simulink model "Template"  (Simulink 7.3)
settings: Solver=ode45  StartTime=0.0  StopTime=10.0  RelTol=1e-3
libraries: marine_gnc x4, dspmtrx3 x2, simulink x2, simulink_extras x1
settings Model: Creator=mcl  LastModifiedBy=mcl

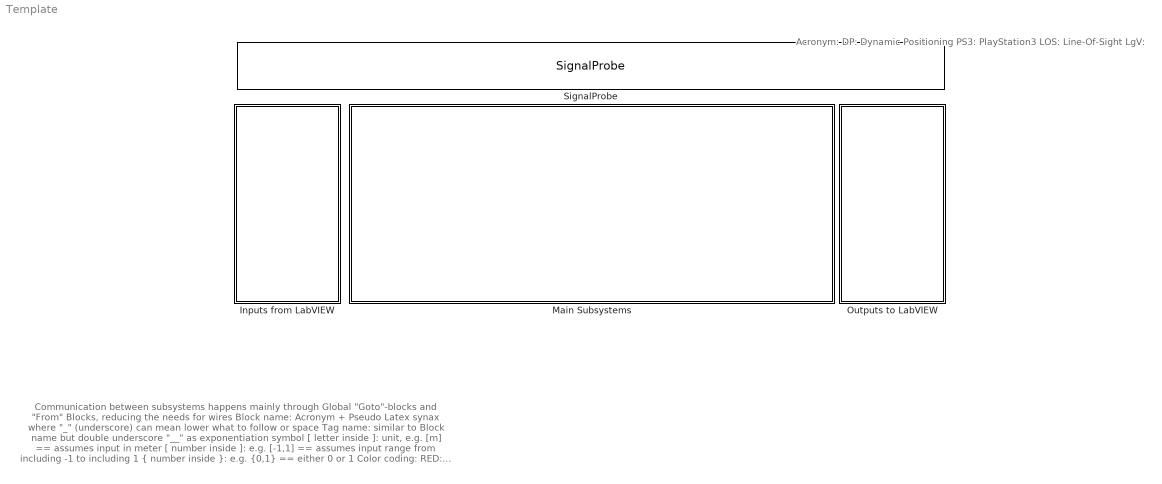
== system Template ==
  note: Communication between subsystems happens mainly through Global "Goto"-blocks and "From" Blocks,
      | reducing the needs for wires
      |
      | Block name: Acronym + Pseudo Latex synax where "_" (underscore) can mean lower what to follow or space
      | Tag name: similar to Block name but double underscore "__" as exponentiation symbol
      |
      | [ letter inside ]: unit, e.g. [m] == assumes input in meter
      | [ number inside ]: e.g. [-1,1] == assumes input range from including -1 to including 1
      | { number inside }:  e.g. {0,1} == either 0 or 1
      |
      | Color coding:
      | RED: Sinks (output ports, terminators, to workspace blocks, etc.)
      | GREEN Sources (inputs ports, constants, etc.)
      | CYAN: Memory blocks: Integrators, unit delays, memory, transfer functions, state space blocks, etc
      | GRAY: Logics blocks: Logic action ports, subsystem enable, etc.
      | ORANGE: GOTO blocks
      | MAGENTA: FROM blocks
      | YELLOW: All remaining blocks,
  note: Acronym:
      | DP: Dynamic Positioning
      | PS3: PlayStation3
      | LOS: Line-Of-Sight
      | LgV:
  Inputs from LabVIEW : Subsystem
  Main Subsystems : Subsystem
  Outputs to LabVIEW : Subsystem
  SignalProbe : S-Function  Description=Use this block with SIT.  FunctionName=SignalProbe  Parameters=1  EnableBusSupport=off
      settings: PreSaveFcn=NISIT_ModelVars;
      mask Description: The LabVIEW Simulation Interface Toolkit uses the SignalProbe block to probe the signals in the model. The SignalProbe block must be on the top level of the model hierarchy. You can have only one SignalProbe block per model file. Do not rename the SignalProbe block. Do not change the name of another model block to SignalProbe.

== system Template/Inputs from LabVIEW ==
  Control Input Selector : Constant  Value=0
  Control Mode Selector : Constant  Value=0
  DynamicPositioning : Subsystem
  Enable CSE1 : Constant  Value=0
  Initial eta : Subsystem
  Initial nu : Subsystem
  LOS LgV backstepping II : Subsystem
  Linear Simulator : Subsystem
  Path : Subsystem
  PlayStation3 : Subsystem
  tag scope: Control_Input_Selector=global, Control_Mode_Selector=global, Enable_CSE1=global
  wires:
  Control Mode Selector/1 -> [Control_Mode_Selector]
  Control Input Selector/1 -> [Control_Input_Selector]
  Enable CSE1/1 -> [Enable_CSE1]

== system Template/Main Subsystems ==
  DP control : Subsystem
  Guidance : Subsystem
  Input from SIT : Subsystem
  Subsystem : Subsystem

== system Template/Outputs to LabVIEW ==
  note: Gain blocks in this subsystem, functions as output ports for linking LabVIEW indicators through SIT Connection Manager
  Battery Voltage : Subsystem

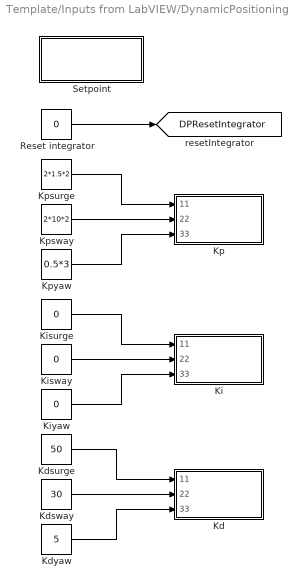
== system Template/Inputs from LabVIEW/DynamicPositioning ==
  Kd : Subsystem
  Kdsurge : Constant  Value=50
  Kdsway : Constant  Value=30
  Kdyaw : Constant  Value=5
  Ki : Subsystem
  Kisurge : Constant  Value=0
  Kisway : Constant  Value=0
  Kiyaw : Constant  Value=0
  Kp : Subsystem
  Kpsurge : Constant  Value=2*1.5*2
  Kpsway : Constant  Value=2*10*2
  Kpyaw : Constant  Value=0.5*3
  Reset integrator : Constant  Value=0
  Setpoint : Subsystem
  tag scope: DPResetIntegrator=global
  wires:
  Reset integrator/1 -> [DPResetIntegrator]
  Kpsurge/1 -> Kp/1(11)
  Kpsway/1 -> Kp/2(22)
  Kpyaw/1 -> Kp/3(33)
  Kdsurge/1 -> Kd/1(11)
  Kdsway/1 -> Kd/2(22)
  Kdyaw/1 -> Kd/3(33)
  Kisurge/1 -> Ki/1(11)
  Kisway/1 -> Ki/2(22)
  Kiyaw/1 -> Ki/3(33)

== system Template/Inputs from LabVIEW/Initial eta ==
  Mux : Mux  Inputs=3
  psi_0 : Constant  Value=0  OutDataType=fixdt(1, 16)  OutScaling=2^0
  x_0 : Constant  Value=0  OutDataType=fixdt(1, 16)  OutScaling=2^0
  y_0 : Constant  Value=0  OutDataType=fixdt(1, 16)  OutScaling=2^0
  eta_0 : Outport  OutDataType=fixdt(1, 16)  OutScaling=2^0
  wires:
  x_0/1 -> Mux/1
  y_0/1 -> Mux/2
  psi_0/1 -> Mux/3
  Mux/1 -> eta_0/1

== system Template/Inputs from LabVIEW/Initial nu ==
  Mux : Mux  Inputs=3
  r_0 : Constant  Value=0  OutDataType=fixdt(1, 16)  OutScaling=2^0
  u_0 : Constant  Value=0  OutDataType=fixdt(1, 16)  OutScaling=2^0
  v_0 : Constant  Value=0  OutDataType=fixdt(1, 16)  OutScaling=2^0
  nu_0 : Outport  OutDataType=fixdt(1, 16)  OutScaling=2^0
  wires:
  u_0/1 -> Mux/1
  v_0/1 -> Mux/2
  r_0/1 -> Mux/3
  Mux/1 -> nu_0/1

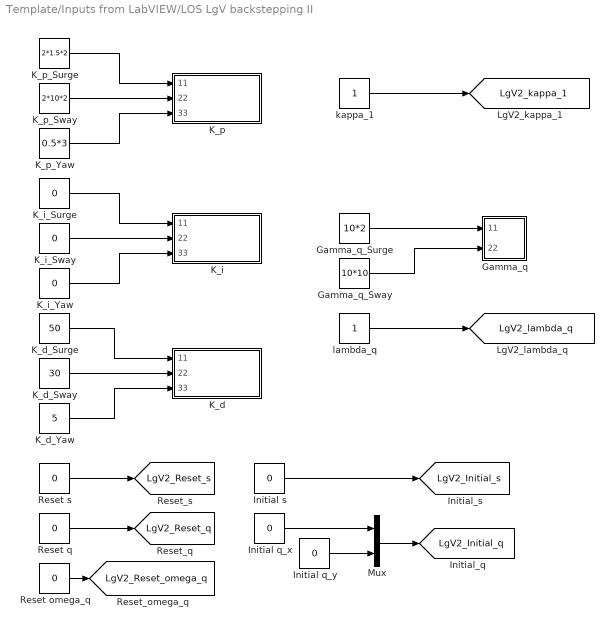
== system Template/Inputs from LabVIEW/LOS LgV backstepping II ==
  Gamma_q : Subsystem
  Gamma_q_Surge : Constant  Value=10*2
  Gamma_q_Sway : Constant  Value=10*10
  Initial q_x : Constant  Value=0  OutDataType=fixdt(1, 16)  OutScaling=2^0
  Initial q_y : Constant  Value=0  OutDataType=fixdt(1, 16)  OutScaling=2^0
  Initial s : Constant  Value=0  OutDataType=fixdt(1, 16)  OutScaling=2^0
  K_d : Subsystem
  K_d_Surge : Constant  Value=50
  K_d_Sway : Constant  Value=30
  K_d_Yaw : Constant  Value=5
  K_i : Subsystem
  K_i_Surge : Constant  Value=0
  K_i_Sway : Constant  Value=0
  K_i_Yaw : Constant  Value=0
  K_p : Subsystem
  K_p_Surge : Constant  Value=2*1.5*2
  K_p_Sway : Constant  Value=2*10*2
  K_p_Yaw : Constant  Value=0.5*3
  Mux : Mux  Inputs=2
  Reset omega_q : Constant  Value=0
  Reset q : Constant  Value=0
  Reset s : Constant  Value=0
  kappa_1 : Constant
  lambda_q : Constant
  tag scope: LgV2_Initial_q=global, LgV2_Initial_s=global, LgV2_Reset_omega_q=global, LgV2_Reset_q=global, LgV2_Reset_s=global, LgV2_kappa_1=global, LgV2_lambda_q=global
  wires:
  K_p_Surge/1 -> K_p/1(11)
  K_p_Sway/1 -> K_p/2(22)
  K_p_Yaw/1 -> K_p/3(33)
  K_d_Surge/1 -> K_d/1(11)
  K_d_Sway/1 -> K_d/2(22)
  K_d_Yaw/1 -> K_d/3(33)
  K_i_Surge/1 -> K_i/1(11)
  K_i_Sway/1 -> K_i/2(22)
  K_i_Yaw/1 -> K_i/3(33)
  Gamma_q_Surge/1 -> Gamma_q/1(11)
  Gamma_q_Sway/1 -> Gamma_q/2(22)
  kappa_1/1 -> [LgV2_kappa_1]
  lambda_q/1 -> [LgV2_lambda_q]
  Initial q_x/1 -> Mux/1
  Initial q_y/1 -> Mux/2
  Reset s/1 -> [LgV2_Reset_s]
  Reset q/1 -> [LgV2_Reset_q]
  Initial s/1 -> [LgV2_Initial_s]
  Mux/1 -> [LgV2_Initial_q]
  Reset omega_q/1 -> [LgV2_Reset_omega_q]

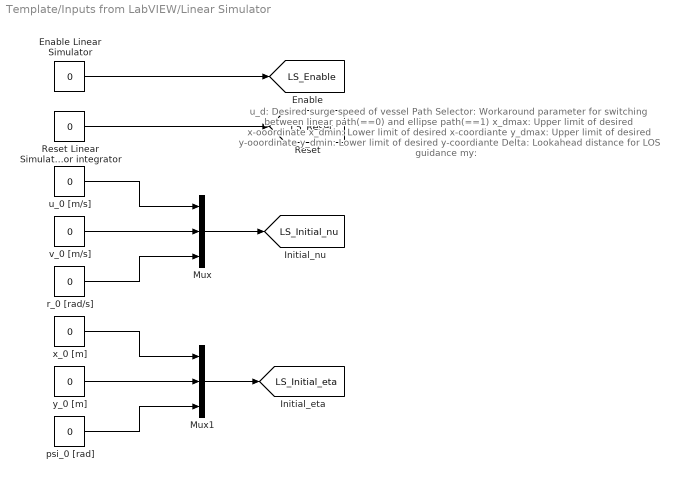
== system Template/Inputs from LabVIEW/Linear Simulator ==
  note: u_d: Desired surge speed of vessel
      | Path Selector: Workaround parameter for switching between linear path(==0) and ellipse path(==1)
      | x_dmax: Upper limit of desired x-ooordinate
      | x_dmin: Lower limit of desired x-coordiante
      | y_dmax: Upper limit of desired y-ooordinate
      | y_dmin: Lower limit of desired y-coordiante
      | Delta: Lookahead distance for LOS guidance
      | my:
  Enable Linear Simulator : Constant  Value=0
  Mux : Mux  Inputs=3
  Mux1 : Mux  Inputs=3
  Reset Linear Simulator integrator : Constant  Value=0
  psi_0 [rad] : Constant  Value=0  OutDataType=fixdt(1, 16)  OutScaling=2^0
  r_0 [rad/s] : Constant  Value=0  OutDataType=fixdt(1, 16)  OutScaling=2^0
  u_0 [m/s] : Constant  Value=0  OutDataType=fixdt(1, 16)  OutScaling=2^0
  v_0 [m/s] : Constant  Value=0  OutDataType=fixdt(1, 16)  OutScaling=2^0
  x_0 [m] : Constant  Value=0  OutDataType=fixdt(1, 16)  OutScaling=2^0
  y_0 [m] : Constant  Value=0  OutDataType=fixdt(1, 16)  OutScaling=2^0
  tag scope: LS_Enable=global, LS_Initial_eta=global, LS_Initial_nu=global, LS_Reset=global
  wires:
  Enable Linear Simulator/1 -> [LS_Enable]
  Reset Linear Simulator integrator/1 -> [LS_Reset]
  Mux/1 -> [LS_Initial_nu]
  r_0 [rad/s]/1 -> Mux/3
  v_0 [m/s]/1 -> Mux/2
  u_0 [m/s]/1 -> Mux/1
  Mux1/1 -> [LS_Initial_eta]
  psi_0 [rad]/1 -> Mux1/3
  y_0 [m]/1 -> Mux1/2
  x_0 [m]/1 -> Mux1/1

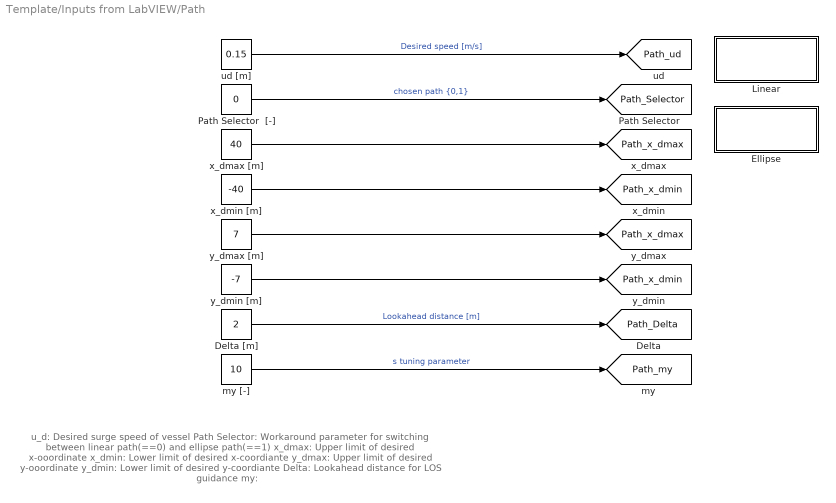
== system Template/Inputs from LabVIEW/Path ==
  note: u_d: Desired surge speed of vessel
      | Path Selector: Workaround parameter for switching between linear path(==0) and ellipse path(==1)
      | x_dmax: Upper limit of desired x-ooordinate
      | x_dmin: Lower limit of desired x-coordiante
      | y_dmax: Upper limit of desired y-ooordinate
      | y_dmin: Lower limit of desired y-coordiante
      | Delta: Lookahead distance for LOS guidance
      | my:
  Delta [m] : Constant  Value=2  OutDataType=fixdt(1, 16)  OutScaling=2^0
  Ellipse : Subsystem
  Linear : Subsystem
  Path Selector  [-] : Constant  Value=0
  my [-] : Constant  Value=10  OutDataType=fixdt(1, 16)  OutScaling=2^0
  ud [m] : Constant  Value=0.15  OutDataType=fixdt(1, 16)  OutScaling=2^0
  x_dmax [m] : Constant  Value=40
  x_dmin [m] : Constant  Value=-40
  y_dmax [m] : Constant  Value=7
  y_dmin [m] : Constant  Value=-7
  tag scope: Path_Delta=global, Path_Selector=global, Path_my=global, Path_ud=global, Path_x_dmax=global, Path_x_dmin=global
  wires:
  ud [m]/1 -> [Path_ud]  "Desired speed [m/s]"
  Delta [m]/1 -> [Path_Delta]  "Lookahead distance [m]"
  my [-]/1 -> [Path_my]  "s tuning parameter"
  Path Selector  [-]/1 -> [Path_Selector]  "chosen path {0,1}"
  x_dmax [m]/1 -> [Path_x_dmax]
  x_dmin [m]/1 -> [Path_x_dmin]
  y_dmax [m]/1 -> [Path_x_dmax]
  y_dmin [m]/1 -> [Path_x_dmin]

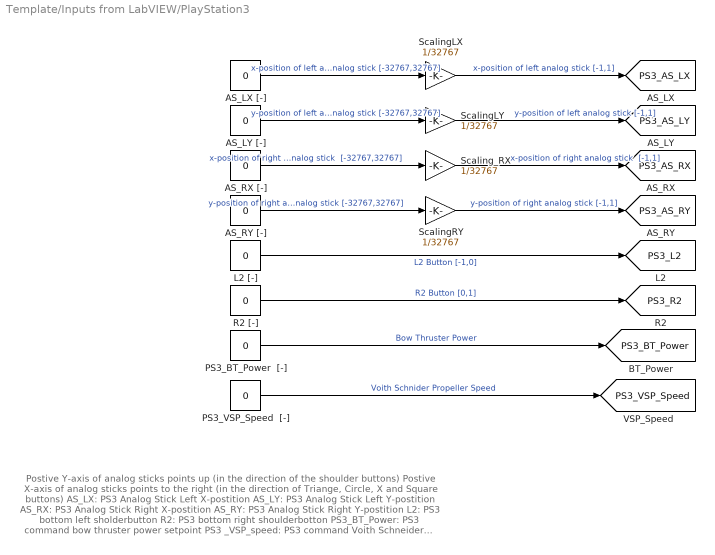
== system Template/Inputs from LabVIEW/PlayStation3 ==
  note: Postive Y-axis of analog sticks points up (in the direction of the shoulder buttons)
      | Postive X-axis of analog sticks points to the right (in the direction of Triange, Circle, X and Square buttons)
      |
      | AS_LX: PS3 Analog Stick Left X-postition
      | AS_LY: PS3 Analog Stick Left Y-postition
      | AS_RX: PS3 Analog Stick Right X-postition
      | AS_RY: PS3 Analog Stick Right Y-postition
      | L2: PS3 bottom left sholderbutton
      | R2: PS3 bottom right shoulderbotton
      | PS3_BT_Power: PS3 command bow thruster power setpoint
      | PS3 _VSP_speed: PS3 command Voith Schneider Propeller speed
  "AS_LX [-] " : Constant  Value=0
  AS_LY [-] : Constant  Value=0
  AS_RX [-] : Constant  Value=0
  AS_RY [-] : Constant  Value=0
  L2 [-] : Constant  Value=0
  PS3_BT_Power  [-] : Constant  Value=0
  PS3_VSP_Speed  [-] : Constant  Value=0
  R2 [-] : Constant  Value=0
  ScalingLX : Gain  Gain=1/32767
  ScalingLY : Gain  Gain=1/32767
  ScalingRY : Gain  Gain=1/32767
  Scaling_RX : Gain  Gain=1/32767
  tag scope: PS3_AS_LX=global, PS3_AS_LY=global, PS3_AS_RX=global, PS3_AS_RY=global, PS3_BT_Power=global, PS3_L2=global, PS3_R2=global, PS3_VSP_Speed=global
  wires:
  PS3_VSP_Speed  [-]/1 -> [PS3_VSP_Speed]  "Voith Schnider Propeller Speed"
  PS3_BT_Power  [-]/1 -> [PS3_BT_Power]  "Bow Thruster Power"
  "AS_LX [-] "/1 -> ScalingLX/1  "x-position of left analog stick [-32767,32767]"
  ScalingLX/1 -> [PS3_AS_LX]  "x-position of left analog stick [-1,1]"
  AS_LY [-]/1 -> ScalingLY/1  "y-position of left analog stick [-32767,32767]"
  ScalingLY/1 -> [PS3_AS_LY]  "y-position of left analog stick [-1,1]"
  AS_RX [-]/1 -> Scaling_RX/1  "x-position of right analog stick  [-32767,32767]"
  Scaling_RX/1 -> [PS3_AS_RX]  "x-position of right analog stick  [-1,1]"
  ScalingRY/1 -> [PS3_AS_RY]  "y-position of right analog stick [-1,1]"
  AS_RY [-]/1 -> ScalingRY/1  "y-position of right analog stick [-32767,32767]"
  L2 [-]/1 -> [PS3_L2]  "L2 Button [-1,0]"
  R2 [-]/1 -> [PS3_R2]  "R2 Button [0,1]"

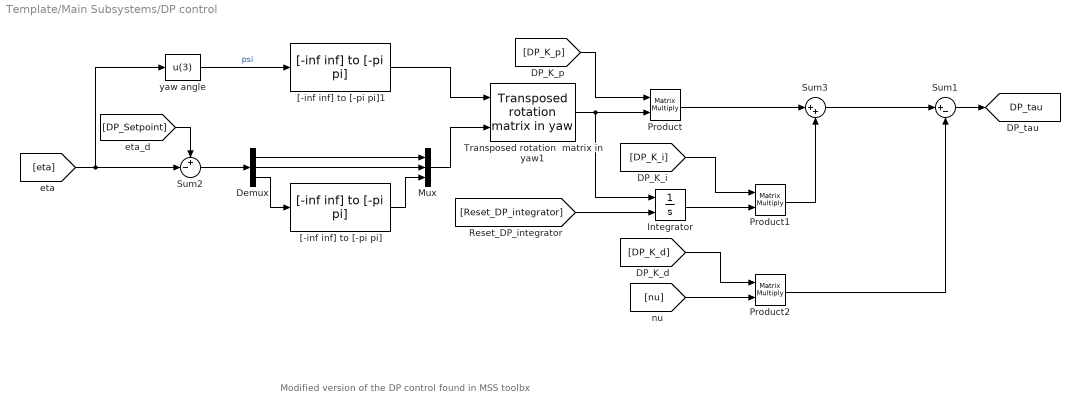
== system Template/Main Subsystems/DP control ==
  note: Modified version of the DP control found in MSS toolbx
  Demux : Demux  Outputs=3
  Integrator : Integrator  ExternalReset=level
  Mux : Mux  Inputs=3
  Product : Product  Multiplication=Matrix(*)  OutDataType=fixdt(1, 16)  OutScaling=2^0  RndMeth=Zero
  Product1 : Product  Multiplication=Matrix(*)  OutDataType=fixdt(1, 16)  OutScaling=2^0  RndMeth=Zero
  Product2 : Product  Multiplication=Matrix(*)  OutDataType=fixdt(1, 16)  OutScaling=2^0  RndMeth=Zero
  Sum1 : Sum  Inputs=|+-  SaturateOnIntegerOverflow=on  InputSameDT=on  OutDataTypeStr=Inherit: Same as first input
  Sum2 : Sum  Inputs=+-|  SaturateOnIntegerOverflow=on  InputSameDT=on  OutDataTypeStr=Inherit: Same as first input
  Sum3 : Sum  Inputs=|++  SaturateOnIntegerOverflow=on  InputSameDT=on  OutDataTypeStr=Inherit: Same as first input
  Transposed rotation  matrix in yaw1 : marine_gnc/Models/ Kinematics/Transposed rotation  matrix in yaw  SystemSampleTime=-1
  "[-inf inf] to [-pi pi]" : marine_gnc/Utilities/Math Operations/[-inf inf] to [-pi pi]  SystemSampleTime=-1
  "[-inf inf] to [-pi pi]1" : marine_gnc/Utilities/Math Operations/[-inf inf] to [-pi pi]  SystemSampleTime=-1
  yaw angle : Fcn  Expr=u(3)
  tag scope: DP_tau=global
  wires:
  Mux/1 -> Transposed rotation  matrix in yaw1/2
  Demux/1 -> Mux/1
  Demux/2 -> Mux/2
  [DP_Setpoint] -> Sum2/1
  Sum1/1 -> [DP_tau]
  [eta] -> yaw angle/1, Sum2/2
  Integrator/1 -> Product1/2
  Sum3/1 -> Sum1/1
  Transposed rotation  matrix in yaw1/1 -> Integrator/1, Product/2
  Sum2/1 -> Demux/1
  [nu] -> Product2/2
  [Reset_DP_integrator] -> Integrator/2
  yaw angle/1 -> "[-inf inf] to [-pi pi]1"/1  "psi"
  "[-inf inf] to [-pi pi]1"/1 -> Transposed rotation  matrix in yaw1/1
  Demux/3 -> "[-inf inf] to [-pi pi]"/1
  "[-inf inf] to [-pi pi]"/1 -> Mux/3
  Product2/1 -> Sum1/2
  Product/1 -> Sum3/1
  Product1/1 -> Sum3/2
  [DP_K_p] -> Product/1
  [DP_K_i] -> Product1/1
  [DP_K_d] -> Product2/1

== system Template/Main Subsystems/Guidance ==
  Line-Of-Sight Path-Following : Subsystem

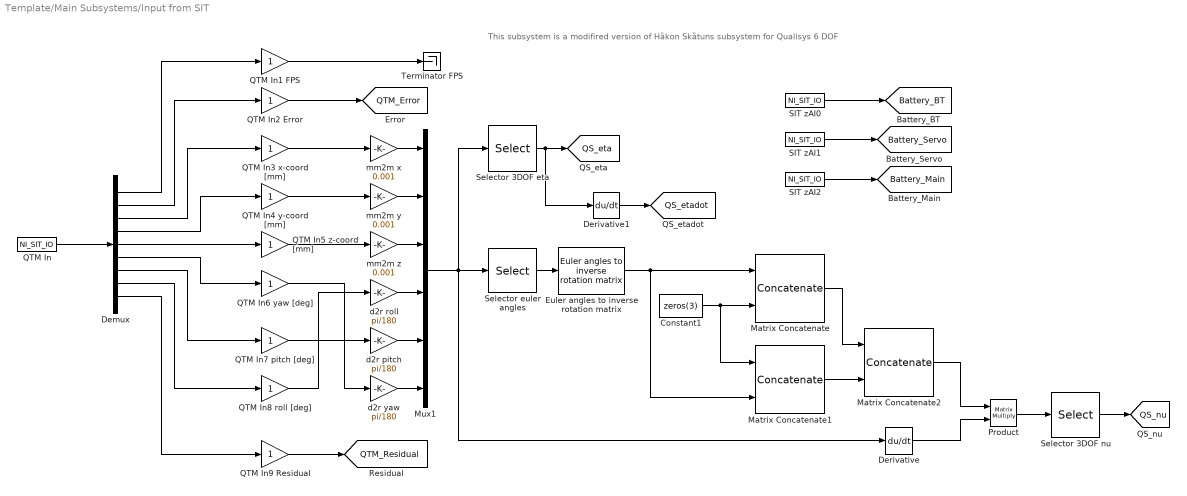
== system Template/Main Subsystems/Input from SIT ==
  note: This subsystem is a modifired version of Håkon Skåtuns subsystem for Qualisys 6 DOF
  Constant1 : Constant  Value=zeros(3)
  Demux : Demux  Outputs=9
  Derivative : Derivative
  Derivative1 : Derivative
  Euler angles to inverse rotation matrix : marine_gnc/Models/ Kinematics/Euler angles to inverse rotation matrix  SystemSampleTime=-1
  Matrix Concatenate : Concatenate  Mode=Multidimensional array
  Matrix Concatenate1 : Concatenate  Mode=Multidimensional array
  Matrix Concatenate2 : Concatenate  Mode=Multidimensional array  ConcatenateDimension=2
  Mux1 : Mux  Inputs=6
  Product : Product  Multiplication=Matrix(*)  RndMeth=Zero
  QTM In : S-Function  Priority=1  FunctionName=NI_SIT_IO  Parameters=width dtype portnum stime stype btype  EnableBusSupport=off  mask(SIT Inport){portnum=1, width=9, stime=-1, dtype=auto, stype=auto, btype=1}
      mask prompts: portnum "Port number:"; width "Port dimensions (-1 for dynamically sized):"; stime "Sample time (-1 for inherited):"; dtype "Data type:"; stype "Signal type:"; btype "Block type:"
      mask help: Use this inport on any level of nested subsystems to allow the LabVIEW Simulation Interface Toolkit to map hardware to it.
      mask init:
      | NI_SIT_IO_init;
      settings: CopyFcn=NI_SIT_IO_callbacks(1);  DeleteFcn=NI_SIT_IO_callbacks(2);
      mask StyleString: edit,edit,edit,popup(auto|double|single|int8|uint8|int16|uint16|int32|uint32|boolean),popup(auto|real|complex),edit
      mask CallbackString: NI_SIT_IO_callbacks(3);|||NI_SIT_IO_callbacks(4);||
      mask TabNameString: Parameters,Parameters,Parameters,Parameters,Parameters,Parameters
      mask Display:
      | patch([-x x], [-y y], [.90980 .81960 .32156]);
      | plot([0 -x x 0], [rad -y y rad]);
      | fprintf('SIT%d', portnum);
  QTM In1 FPS : Gain  ParameterDataType=fixdt(1, 16)  ParameterScaling=2^0  OutDataType=fixdt(1, 16)  OutScaling=2^0
  QTM In2 Error : Gain  ParameterDataType=fixdt(1, 16)  ParameterScaling=2^0  OutDataType=fixdt(1, 16)  OutScaling=2^0
  QTM In3 x-coord [mm] : Gain  ParameterDataType=fixdt(1, 16)  ParameterScaling=2^0  OutDataType=fixdt(1, 16)  OutScaling=2^0
  QTM In4 y-coord [mm] : Gain  ParameterDataType=fixdt(1, 16)  ParameterScaling=2^0  OutDataType=fixdt(1, 16)  OutScaling=2^0
  QTM In5 z-coord [mm] : Gain  ParameterDataType=fixdt(1, 16)  ParameterScaling=2^0  OutDataType=fixdt(1, 16)  OutScaling=2^0
  QTM In6 yaw [deg] : Gain  ParameterDataType=fixdt(1, 16)  ParameterScaling=2^0  OutDataType=fixdt(1, 16)  OutScaling=2^0
  QTM In7 pitch [deg] : Gain  ParameterDataType=fixdt(1, 16)  ParameterScaling=2^0  OutDataType=fixdt(1, 16)  OutScaling=2^0
  QTM In8 roll [deg] : Gain  ParameterDataType=fixdt(1, 16)  ParameterScaling=2^0  OutDataType=fixdt(1, 16)  OutScaling=2^0
  QTM In9 Residual : Gain  ParameterDataType=fixdt(1, 16)  ParameterScaling=2^0  OutDataType=fixdt(1, 16)  OutScaling=2^0
  SIT zAI0 : S-Function  Priority=2  FunctionName=NI_SIT_IO  Parameters=width dtype portnum stime stype btype  EnableBusSupport=off  mask(SIT Inport){portnum=2, width=-1, stime=-1, dtype=auto, stype=auto, btype=1}
      mask prompts: portnum "Port number:"; width "Port dimensions (-1 for dynamically sized):"; stime "Sample time (-1 for inherited):"; dtype "Data type:"; stype "Signal type:"; btype "Block type:"
      mask help: Use this inport on any level of nested subsystems to allow the LabVIEW Simulation Interface Toolkit to map hardware to it.
      mask init:
      | NI_SIT_IO_init;
      settings: CopyFcn=NI_SIT_IO_callbacks(1);  DeleteFcn=NI_SIT_IO_callbacks(2);
      mask StyleString: edit,edit,edit,popup(auto|double|single|int8|uint8|int16|uint16|int32|uint32|boolean),popup(auto|real|complex),edit
      mask CallbackString: NI_SIT_IO_callbacks(3);|||NI_SIT_IO_callbacks(4);||
      mask TabNameString: Parameters,Parameters,Parameters,Parameters,Parameters,Parameters
      mask Display:
      | patch([-x x], [-y y], [.90980 .81960 .32156]);
      | plot([0 -x x 0], [rad -y y rad]);
      | fprintf('SIT%d', portnum);
  SIT zAI1 : S-Function  Priority=3  FunctionName=NI_SIT_IO  Parameters=width dtype portnum stime stype btype  EnableBusSupport=off  mask(SIT Inport){portnum=3, width=-1, stime=-1, dtype=auto, stype=auto, btype=1}
      mask prompts: portnum "Port number:"; width "Port dimensions (-1 for dynamically sized):"; stime "Sample time (-1 for inherited):"; dtype "Data type:"; stype "Signal type:"; btype "Block type:"
      mask help: Use this inport on any level of nested subsystems to allow the LabVIEW Simulation Interface Toolkit to map hardware to it.
      mask init:
      | NI_SIT_IO_init;
      settings: CopyFcn=NI_SIT_IO_callbacks(1);  DeleteFcn=NI_SIT_IO_callbacks(2);
      mask StyleString: edit,edit,edit,popup(auto|double|single|int8|uint8|int16|uint16|int32|uint32|boolean),popup(auto|real|complex),edit
      mask CallbackString: NI_SIT_IO_callbacks(3);|||NI_SIT_IO_callbacks(4);||
      mask TabNameString: Parameters,Parameters,Parameters,Parameters,Parameters,Parameters
      mask Display:
      | patch([-x x], [-y y], [.90980 .81960 .32156]);
      | plot([0 -x x 0], [rad -y y rad]);
      | fprintf('SIT%d', portnum);
  SIT zAI2 : S-Function  Priority=4  FunctionName=NI_SIT_IO  Parameters=width dtype portnum stime stype btype  EnableBusSupport=off  mask(SIT Inport){portnum=4, width=-1, stime=-1, dtype=auto, stype=auto, btype=1}
      mask prompts: portnum "Port number:"; width "Port dimensions (-1 for dynamically sized):"; stime "Sample time (-1 for inherited):"; dtype "Data type:"; stype "Signal type:"; btype "Block type:"
      mask help: Use this inport on any level of nested subsystems to allow the LabVIEW Simulation Interface Toolkit to map hardware to it.
      mask init:
      | NI_SIT_IO_init;
      settings: CopyFcn=NI_SIT_IO_callbacks(1);  DeleteFcn=NI_SIT_IO_callbacks(2);
      mask StyleString: edit,edit,edit,popup(auto|double|single|int8|uint8|int16|uint16|int32|uint32|boolean),popup(auto|real|complex),edit
      mask CallbackString: NI_SIT_IO_callbacks(3);|||NI_SIT_IO_callbacks(4);||
      mask TabNameString: Parameters,Parameters,Parameters,Parameters,Parameters,Parameters
      mask Display:
      | patch([-x x], [-y y], [.90980 .81960 .32156]);
      | plot([0 -x x 0], [rad -y y rad]);
      | fprintf('SIT%d', portnum);
  Selector 3DOF eta : Selector  InputPortWidth=6  IndexOptions=Index vector (dialog)  Indices=[1 2 6]  OutputSizes=1
  Selector 3DOF nu : Selector  InputPortWidth=6  IndexOptions=Index vector (dialog)  Indices=[1 2 6]  OutputSizes=1
  Selector euler angles : Selector  InputPortWidth=6  IndexOptions=Index vector (dialog)  Indices=[4 5 6]  OutputSizes=1
  Terminator FPS : Terminator
  d2r pitch : Gain  Gain=pi/180  ParameterDataType=fixdt(1, 16)  ParameterScaling=2^0  OutDataType=fixdt(1, 16)  OutScaling=2^0
  d2r roll : Gain  Gain=pi/180  ParameterDataType=fixdt(1, 16)  ParameterScaling=2^0  OutDataType=fixdt(1, 16)  OutScaling=2^0
  d2r yaw : Gain  Gain=pi/180  ParameterDataType=fixdt(1, 16)  ParameterScaling=2^0  OutDataType=fixdt(1, 16)  OutScaling=2^0
  mm2m x : Gain  Gain=0.001
  mm2m y : Gain  Gain=0.001
  mm2m z : Gain  Gain=0.001
  tag scope: Battery_BT=global, Battery_Main=global, Battery_Servo=global, QS_eta=global, QS_etadot=global, QS_nu=global, QTM_Error=global, QTM_Residual=global
  wires:
  Mux1/1 -> Selector euler angles/1, Derivative/1, Selector 3DOF eta/1
  Selector 3DOF eta/1 -> Derivative1/1, [QS_eta]
  Euler angles to inverse rotation matrix/1 -> Matrix Concatenate/1, Matrix Concatenate1/2
  Matrix Concatenate/1 -> Matrix Concatenate2/1
  Matrix Concatenate1/1 -> Matrix Concatenate2/2
  Matrix Concatenate2/1 -> Product/1
  Derivative/1 -> Product/2
  Constant1/1 -> Matrix Concatenate/2, Matrix Concatenate1/1
  mm2m z/1 -> Mux1/3
  mm2m y/1 -> Mux1/2
  mm2m x/1 -> Mux1/1
  d2r yaw/1 -> Mux1/6
  d2r pitch/1 -> Mux1/5
  d2r roll/1 -> Mux1/4
  Selector euler angles/1 -> Euler angles to inverse rotation matrix/1
  Product/1 -> Selector 3DOF nu/1
  Selector 3DOF nu/1 -> [QS_nu]
  QTM In1 FPS/1 -> Terminator FPS/1
  QTM In2 Error/1 -> [QTM_Error]
  QTM In9 Residual/1 -> [QTM_Residual]
  QTM In/1 -> Demux/1
  Demux/1 -> QTM In1 FPS/1
  Demux/2 -> QTM In2 Error/1
  Demux/3 -> QTM In3 x-coord [mm]/1
  Demux/4 -> QTM In4 y-coord [mm]/1
  Demux/5 -> QTM In5 z-coord [mm]/1
  Demux/6 -> QTM In6 yaw [deg]/1
  Demux/7 -> QTM In7 pitch [deg]/1
  Demux/8 -> QTM In8 roll [deg]/1
  Demux/9 -> QTM In9 Residual/1
  QTM In3 x-coord [mm]/1 -> mm2m x/1
  QTM In4 y-coord [mm]/1 -> mm2m y/1
  QTM In5 z-coord [mm]/1 -> mm2m z/1
  QTM In7 pitch [deg]/1 -> d2r pitch/1
  QTM In6 yaw [deg]/1 -> d2r yaw/1
  QTM In8 roll [deg]/1 -> d2r roll/1
  Derivative1/1 -> [QS_etadot]
  SIT zAI0/1 -> [Battery_BT]
  SIT zAI1/1 -> [Battery_Servo]
  SIT zAI2/1 -> [Battery_Main]

== system Template/Main Subsystems/Subsystem ==

== system Template/Outputs to LabVIEW/Battery Voltage ==
  note: Main battery is multipled by 2, since the voltage is halfed at measuring point
  Battery Bow Thruster : Gain  ParameterDataType=fixdt(1, 16)  ParameterScaling=2^0  OutDataType=fixdt(1, 16)  OutScaling=2^0
  Battery Main : Gain  Gain=2  ParameterDataType=fixdt(1, 16)  ParameterScaling=2^0  OutDataType=fixdt(1, 16)  OutScaling=2^0
  Battery Servo : Gain  ParameterDataType=fixdt(1, 16)  ParameterScaling=2^0  OutDataType=fixdt(1, 16)  OutScaling=2^0
  Terminator Bow Thruster Battery : Terminator
  Terminator Main Battery : Terminator
  Terminator Servo Battery : Terminator
  wires:
  [Battery_BT] -> Battery Bow Thruster/1
  Battery Bow Thruster/1 -> Terminator Bow Thruster Battery/1
  [Battery_Servo] -> Battery Servo/1
  Battery Servo/1 -> Terminator Servo Battery/1
  [Battery_Main] -> Battery Main/1
  Battery Main/1 -> Terminator Main Battery/1

== system Template/Inputs from LabVIEW/DynamicPositioning/Kd ==
  note: Creating 3x3 diagonal matrix
  11 : Inport
  22 : Inport  Port=2
  33 : Inport  Port=3
  {12..13,21,23,31..32} (6 alike) : Constant  Value=0
  Mux : Mux  Inputs=9
  "[3x3]" : Reshape  OutputDimensionality=Customize  OutputDimensions=[3,3]
  tag scope: DPKd=global
  wires:
  "[3x3]"/1 -> [DPKd]
  33/1 -> Mux/9
  23/1 -> Mux/8
  13/1 -> Mux/7
  32/1 -> Mux/6
  22/1 -> Mux/5
  12/1 -> Mux/4
  31/1 -> Mux/3
  21/1 -> Mux/2
  11/1 -> Mux/1
  Mux/1 -> "[3x3]"/1

== system Template/Inputs from LabVIEW/DynamicPositioning/Ki ==
  note: Creating 3x3 diagonal matrix
  11 : Inport
  22 : Inport  Port=2
  33 : Inport  Port=3
  {12..13,21,23,31..32} (6 alike) : Constant  Value=0
  Mux : Mux  Inputs=9
  "[3x3]" : Reshape  OutputDimensionality=Customize  OutputDimensions=[3,3]
  tag scope: DPKi=global
  wires:
  "[3x3]"/1 -> [DPKi]
  33/1 -> Mux/9
  23/1 -> Mux/8
  13/1 -> Mux/7
  32/1 -> Mux/6
  22/1 -> Mux/5
  12/1 -> Mux/4
  31/1 -> Mux/3
  21/1 -> Mux/2
  11/1 -> Mux/1
  Mux/1 -> "[3x3]"/1

== system Template/Inputs from LabVIEW/DynamicPositioning/Kp ==
  note: Creating 3x3 diagonal matrix
  11 : Inport
  22 : Inport  Port=2
  33 : Inport  Port=3
  {12..13,21,23,31..32} (6 alike) : Constant  Value=0
  Mux : Mux  Inputs=9
  "[3x3]" : Reshape  OutputDimensionality=Customize  OutputDimensions=[3,3]
  tag scope: DPKp=global
  wires:
  Mux/1 -> "[3x3]"/1
  11/1 -> Mux/1
  21/1 -> Mux/2
  31/1 -> Mux/3
  12/1 -> Mux/4
  22/1 -> Mux/5
  32/1 -> Mux/6
  13/1 -> Mux/7
  23/1 -> Mux/8
  33/1 -> Mux/9
  "[3x3]"/1 -> [DPKp]

== system Template/Inputs from LabVIEW/DynamicPositioning/Setpoint ==
  " yd [m]" : Constant  Value=0
  Degrees to Radians : simulink_extras/Transformations/Degrees to Radians  SystemSampleTime=-1
  Mux : Mux  Inputs=3
  psid [deg] : Constant  Value=0
  xd [m] : Constant  Value=0
  tag scope: DPSetpoint=global
  wires:
  Degrees to Radians/1 -> Mux/3
  psid [deg]/1 -> Degrees to Radians/1
  " yd [m]"/1 -> Mux/2
  xd [m]/1 -> Mux/1
  Mux/1 -> [DPSetpoint]

== system Template/Inputs from LabVIEW/LOS LgV backstepping II/Gamma_q ==
  11 : Inport
  22 : Inport  Port=2
  12 : Constant  Value=0
  21 : Constant  Value=0
  Mux : Mux
  "[2x2]" : Reshape  OutputDimensionality=Customize  OutputDimensions=[2,2]
  tag scope: LgV2_Gamma_q=global
  wires:
  Mux/1 -> "[2x2]"/1
  11/1 -> Mux/1
  21/1 -> Mux/2
  12/1 -> Mux/3
  22/1 -> Mux/4
  "[2x2]"/1 -> [LgV2_Gamma_q]

== system Template/Inputs from LabVIEW/LOS LgV backstepping II/K_d ==
  note: Creating 3x3 diagonal matrix
  11 : Inport
  22 : Inport  Port=2
  33 : Inport  Port=3
  {12..13,21,23,31..32} (6 alike) : Constant  Value=0
  Mux : Mux  Inputs=9
  "[3x3]" : Reshape  OutputDimensionality=Customize  OutputDimensions=[3,3]
  tag scope: LgV2_K_d=global
  wires:
  "[3x3]"/1 -> [LgV2_K_d]
  33/1 -> Mux/9
  23/1 -> Mux/8
  13/1 -> Mux/7
  32/1 -> Mux/6
  22/1 -> Mux/5
  12/1 -> Mux/4
  31/1 -> Mux/3
  21/1 -> Mux/2
  11/1 -> Mux/1
  Mux/1 -> "[3x3]"/1

== system Template/Inputs from LabVIEW/LOS LgV backstepping II/K_i ==
  note: Creating 3x3 diagonal matrix
  11 : Inport
  22 : Inport  Port=2
  33 : Inport  Port=3
  {12..13,21,23,31..32} (6 alike) : Constant  Value=0
  Mux : Mux  Inputs=9
  "[3x3]" : Reshape  OutputDimensionality=Customize  OutputDimensions=[3,3]
  tag scope: LgV2_K_i=global
  wires:
  "[3x3]"/1 -> [LgV2_K_i]
  33/1 -> Mux/9
  23/1 -> Mux/8
  13/1 -> Mux/7
  32/1 -> Mux/6
  22/1 -> Mux/5
  12/1 -> Mux/4
  31/1 -> Mux/3
  21/1 -> Mux/2
  11/1 -> Mux/1
  Mux/1 -> "[3x3]"/1

== system Template/Inputs from LabVIEW/LOS LgV backstepping II/K_p ==
  note: Creating 3x3 diagonal matrix
  11 : Inport
  22 : Inport  Port=2
  33 : Inport  Port=3
  {12..13,21,23,31..32} (6 alike) : Constant  Value=0
  Mux : Mux  Inputs=9
  "[3x3]" : Reshape  OutputDimensionality=Customize  OutputDimensions=[3,3]
  tag scope: LgV2_K_p=global
  wires:
  Mux/1 -> "[3x3]"/1
  11/1 -> Mux/1
  21/1 -> Mux/2
  31/1 -> Mux/3
  12/1 -> Mux/4
  22/1 -> Mux/5
  32/1 -> Mux/6
  13/1 -> Mux/7
  23/1 -> Mux/8
  33/1 -> Mux/9
  "[3x3]"/1 -> [LgV2_K_p]

== system Template/Inputs from LabVIEW/Path/Ellipse ==
  note: origin_x: ellipse origin x-coordinate
      | origin_y: ellipse origin y-coordinate
      | r_x: ellipse radius x-direction
      | r_y: ellipse radius y-direction
      | k: step scaling factor of path parameter
  k [-] : Constant  Value=pi/180*2  OutDataType=fixdt(1, 16)  OutScaling=2^0
  origin_x [m] : Constant  Value=4.5  OutDataType=fixdt(1, 16)  OutScaling=2^0
  origo_y [m] : Constant  Value=0  OutDataType=fixdt(1, 16)  OutScaling=2^0
  r_x [m] : Constant  Value=5.5  OutDataType=fixdt(1, 16)  OutScaling=2^0
  r_y [m] : Constant  Value=2  OutDataType=fixdt(1, 16)  OutScaling=2^0
  tag scope: PathE_k=global, PathE_origin_x=global, PathE_origin_y=global, PathE_r_x=global, PathE_r_y=global
  wires:
  origin_x [m]/1 -> [PathE_origin_x]  "x-coord. origin ellipse path [m]"
  origo_y [m]/1 -> [PathE_origin_y]  "y-coord. origin ellipse path [m]"
  r_x [m]/1 -> [PathE_r_x]  "radius ellipse path x-axis [m]"
  r_y [m]/1 -> [PathE_r_y]  "radius ellipse path y-axis [m]"
  k [-]/1 -> [PathE_k]  "step scaling factor ellipse path [-]"

== system Template/Inputs from LabVIEW/Path/Linear ==
  note: x_1: reference way-point x-coordinate
      | y_1: reference way-point y-coordinate
      | x_2: direction way-point x-coordinate
      | y_2: direction way-point y-coordinate
  x_1 [m] : Constant  Value=0  OutDataType=fixdt(1, 16)  OutScaling=2^0
  x_2 [m] : Constant  Value=5.5  OutDataType=fixdt(1, 16)  OutScaling=2^0
  y_1 [m] : Constant  Value=0  OutDataType=fixdt(1, 16)  OutScaling=2^0
  y_2 [m] : Constant  Value=2  OutDataType=fixdt(1, 16)  OutScaling=2^0
  tag scope: PathL_x_1=global, PathL_x_2=global, PathL_y_1=global, PathL_y_2=global
  wires:
  x_1 [m]/1 -> [PathL_x_1]  "x-coord. reference point path [m]"
  y_1 [m]/1 -> [PathL_y_1]  "y-coord, reference point path [m]"
  x_2 [m]/1 -> [PathL_x_2]  "x-coord, direction point path [m]"
  y_2 [m]/1 -> [PathL_y_2]  "y-coord, direction point path [m]"

== system Template/Main Subsystems/Guidance/Line-Of-Sight Path-Following ==
  Path : Subsystem

== system Template/Main Subsystems/Guidance/Line-Of-Sight Path-Following/Path ==
  note: Path Selector == 1: Straight path
      | Path Selector == 0: Ellipse path
  Ellipse path : Subsystem
  Path Selector : Constant  Value=0
  Path Switch workaround : Subsystem
  Straight path : Subsystem
  saturation : Subsystem
  p_d^s : Outport
  p_d^s^2 : Outport  Port=2
  p_d^s^3 : Outport  Port=3
  p_d : Outport  Port=4
  |p_d^s| : Outport  Port=5
  path : Outport  Port=6
  wires:
  Path Switch workaround/5(|p_d^s|) -> |p_d^s|/1
  Path Switch workaround/4(p_d^s^3) -> p_d^s^3/1
  Path Switch workaround/3(p_d^s^2) -> p_d^s^2/1
  Path Switch workaround/2(p_d^s) -> p_d^s/1
  Path Switch workaround/1(p_d) -> saturation/1(p_d)
  saturation/1(sat_p_d) -> p_d/1
  Ellipse path/5(|p_d^s|) -> Path Switch workaround/11(|p_d^s| Ellipse path)
  Ellipse path/4(p_d^s^3) -> Path Switch workaround/10(p_d^s^2 Ellipse path)
  Ellipse path/3(p_d^s^2) -> Path Switch workaround/9(p_d^s^3 Ellipse path)
  Ellipse path/2(p_d^s) -> Path Switch workaround/8(p_d^s Ellipse path)
  Ellipse path/1(p_d) -> Path Switch workaround/7(p_d Ellipse path)
  Straight path/4(|p_d^s|) -> Path Switch workaround/6(|p_d^s| Straight path)  "|p_d^s|"
  Straight path/3(p_d^s^3) -> Path Switch workaround/5(p_d^s^2 Straight path)  "p_d^s^3"
  Straight path/2(p_d^s^2) -> Path Switch workaround/4(p_d^s^3 Straight path)  "p_d^s^2"
  Straight path/1(p_d^s) -> Path Switch workaround/3(p_d^s Straight path)  "p_d^s"
  ? -> Path Switch workaround/2(p_d Straight path)  "p_d"
  Path Selector/1 -> path/1, Path Switch workaround/1(Path Selector)  "chosen path"

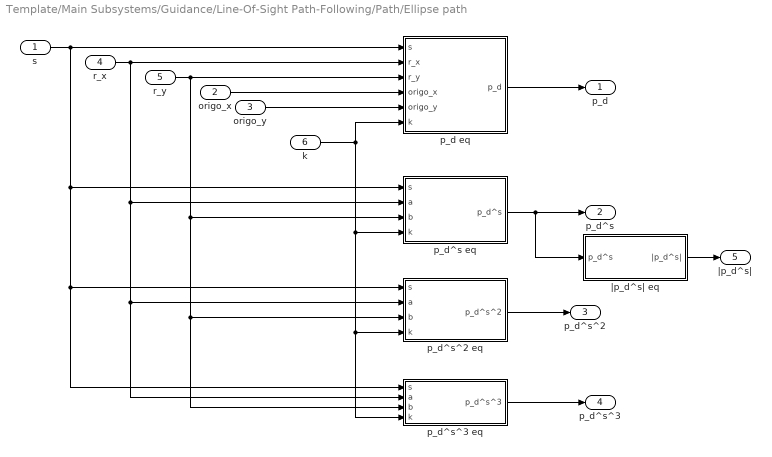
== system Template/Main Subsystems/Guidance/Line-Of-Sight Path-Following/Path/Ellipse path ==
  s : Inport
  origo_x : Inport  Port=2
  origo_y : Inport  Port=3
  r_x : Inport  Port=4
  r_y : Inport  Port=5
  k : Inport  Port=6
  p_d eq : Subsystem
  p_d^s eq : Subsystem
  p_d^s^2 eq : Subsystem
  p_d^s^3 eq : Subsystem
  |p_d^s| eq : Subsystem
  p_d : Outport
  p_d^s : Outport  Port=2
  p_d^s^2 : Outport  Port=3
  p_d^s^3 : Outport  Port=4
  |p_d^s| : Outport  Port=5
  wires:
  k/1 -> p_d^s^3 eq/4(k), p_d^s^2 eq/4(k), p_d^s eq/4(k), p_d eq/6(k)
  origo_y/1 -> p_d eq/5(origo_y)
  origo_x/1 -> p_d eq/4(origo_x)
  r_y/1 -> p_d^s eq/3(b), p_d^s^3 eq/3(b), p_d^s^2 eq/3(b), p_d eq/3(r_y)
  r_x/1 -> p_d^s^3 eq/2(a), p_d^s^2 eq/2(a), p_d^s eq/2(a), p_d eq/2(r_x)
  s/1 -> p_d^s^3 eq/1(s), p_d^s^2 eq/1(s), p_d^s eq/1(s), p_d eq/1(s)
  p_d eq/1(p_d) -> p_d/1
  |p_d^s| eq/1(|p_d^s|) -> |p_d^s|/1
  p_d^s^2 eq/1(p_d^s^2) -> p_d^s^2/1
  p_d^s^3 eq/1(p_d^s^3) -> p_d^s^3/1
  p_d^s eq/1(p_d^s) -> p_d^s/1, |p_d^s| eq/1(p_d^s)

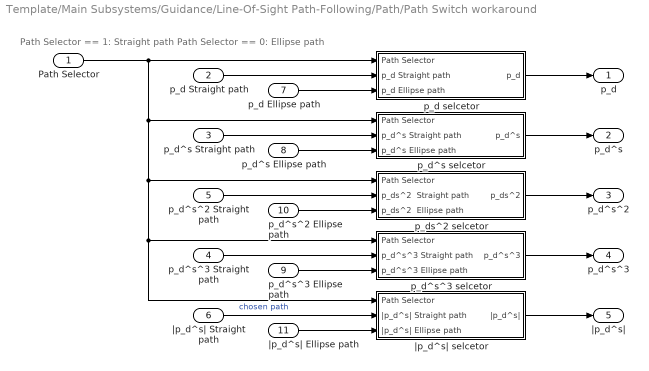
== system Template/Main Subsystems/Guidance/Line-Of-Sight Path-Following/Path/Path Switch workaround ==
  note: Path Selector == 1: Straight path
      | Path Selector == 0: Ellipse path
  Path Selector : Inport  OutDataType=fixdt(1, 16)  OutScaling=2^0
  p_d Straight path : Inport  Port=2  OutDataType=fixdt(1, 16)  OutScaling=2^0
  p_d^s Straight path : Inport  Port=3  OutDataType=fixdt(1, 16)  OutScaling=2^0
  p_d^s^3 Straight path : Inport  Port=4  OutDataType=fixdt(1, 16)  OutScaling=2^0
  p_d^s^2 Straight path : Inport  Port=5  OutDataType=fixdt(1, 16)  OutScaling=2^0
  |p_d^s| Straight path : Inport  Port=6  OutDataType=fixdt(1, 16)  OutScaling=2^0
  p_d Ellipse path : Inport  Port=7  OutDataType=fixdt(1, 16)  OutScaling=2^0
  p_d^s Ellipse path : Inport  Port=8  OutDataType=fixdt(1, 16)  OutScaling=2^0
  p_d^s^3 Ellipse path : Inport  Port=9  OutDataType=fixdt(1, 16)  OutScaling=2^0
  p_d^s^2 Ellipse path : Inport  Port=10  OutDataType=fixdt(1, 16)  OutScaling=2^0
  |p_d^s| Ellipse path : Inport  Port=11  OutDataType=fixdt(1, 16)  OutScaling=2^0
  p_d selcetor : Subsystem
  p_d^s selcetor : Subsystem
  p_d^s^3 selcetor : Subsystem
  p_ds^2 selcetor : Subsystem
  |p_d^s| selcetor : Subsystem
  p_d : Outport
  p_d^s : Outport  Port=2
  p_d^s^2 : Outport  Port=3
  p_d^s^3 : Outport  Port=4
  |p_d^s| : Outport  Port=5
  wires:
  |p_d^s| Ellipse path/1 -> |p_d^s| selcetor/3(|p_d^s| Ellipse path)
  |p_d^s| Straight path/1 -> |p_d^s| selcetor/2(|p_d^s| Straight path)
  p_d^s^3 Ellipse path/1 -> p_d^s^3 selcetor/3(p_d^s^3 Ellipse path)
  p_d^s^3 Straight path/1 -> p_d^s^3 selcetor/2(p_d^s^3 Straight path)
  p_d^s^2 Ellipse path/1 -> p_ds^2 selcetor/3(p_ds^2  Ellipse path)
  p_d^s^2 Straight path/1 -> p_ds^2 selcetor/2(p_ds^2  Straight path)
  p_d^s Ellipse path/1 -> p_d^s selcetor/3(p_d^s Ellipse path)
  p_d^s Straight path/1 -> p_d^s selcetor/2(p_d^s Straight path)
  p_d Ellipse path/1 -> p_d selcetor/3(p_d Ellipse path)
  p_d Straight path/1 -> p_d selcetor/2(p_d Straight path)
  Path Selector/1 -> |p_d^s| selcetor/1(Path Selector), p_d^s^3 selcetor/1(Path Selector), p_ds^2 selcetor/1(Path Selector), p_d^s selcetor/1(Path Selector), p_d selcetor/1(Path Selector)  "chosen path"
  |p_d^s| selcetor/1(|p_d^s|) -> |p_d^s|/1
  p_d^s^3 selcetor/1("p_d^s^3 ") -> p_d^s^3/1
  p_ds^2 selcetor/1("p_ds^2 ") -> p_d^s^2/1
  p_d^s selcetor/1(p_d^s) -> p_d^s/1
  p_d selcetor/1(p_d) -> p_d/1

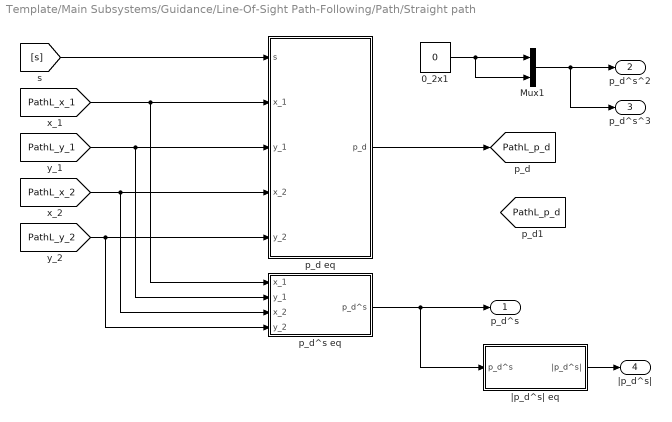
== system Template/Main Subsystems/Guidance/Line-Of-Sight Path-Following/Path/Straight path ==
  0_2x1 : Constant  Value=0  VectorParams1D=off  OutDataType=fixdt(1, 16)  OutScaling=2^0
  Mux1 : Mux  Inputs=2
  p_d eq : Subsystem
  p_d^s eq : Subsystem
  |p_d^s| eq : Subsystem
  p_d^s : Outport
  p_d^s^2 : Outport  Port=2
  p_d^s^3 : Outport  Port=3
  |p_d^s| : Outport  Port=4
  tag scope: PathL_p_d=global
  wires:
  p_d eq/1(p_d) -> [PathL_p_d]
  Mux1/1 -> p_d^s^3/1, p_d^s^2/1
  0_2x1/1 -> Mux1/2, Mux1/1
  [PathL_y_2] -> p_d eq/5(y_2), p_d^s eq/4(y_2)
  [PathL_x_2] -> p_d eq/4(x_2), p_d^s eq/3(x_2)
  [PathL_y_1] -> p_d eq/3(y_1), p_d^s eq/2(y_1)
  [PathL_x_1] -> p_d eq/2(x_1), p_d^s eq/1(x_1)
  [s] -> p_d eq/1(s)
  |p_d^s| eq/1(|p_d^s|) -> |p_d^s|/1
  p_d^s eq/1(p_d^s) -> p_d^s/1, |p_d^s| eq/1(p_d^s)

== system Template/Main Subsystems/Guidance/Line-Of-Sight Path-Following/Path/saturation ==
  p_d : Inport  OutDataType=sfix(16)  OutScaling=2^0
  Demux : Demux  Outputs=2
  Mux1 : Mux  Inputs=2
  Saturation x : simulink/Discontinuities/Saturation Dynamic  SystemSampleTime=-1  OutMin=[]  OutMax=[]  OutDataTypeStr=Inherit: Same as second input  OutDataType=fixdt(1, 16)  OutScaling=2^-10  DoSatur=off
  Saturation y : simulink/Discontinuities/Saturation Dynamic  SystemSampleTime=-1  OutMin=[]  OutMax=[]  OutDataTypeStr=Inherit: Same as second input  OutDataType=fixdt(1, 16)  OutScaling=2^-10  DoSatur=off
  path x_dmax : Constant  Value=10000
  path x_dmin : Constant  Value=-10000
  path y_dmax : Constant  Value=10000
  path y_dmin : Constant  Value=-10000
  sat_p_d : Outport  OutDataType=sfix(16)  OutScaling=2^0
  wires:
  Saturation y/1 -> Mux1/2
  Saturation x/1 -> Mux1/1
  path y_dmax/1 -> Saturation y/1
  path y_dmin/1 -> Saturation y/3
  Demux/2 -> Saturation y/2
  path x_dmin/1 -> Saturation x/3
  path x_dmax/1 -> Saturation x/1
  Demux/1 -> Saturation x/2
  p_d/1 -> Demux/1
  Mux1/1 -> sat_p_d/1

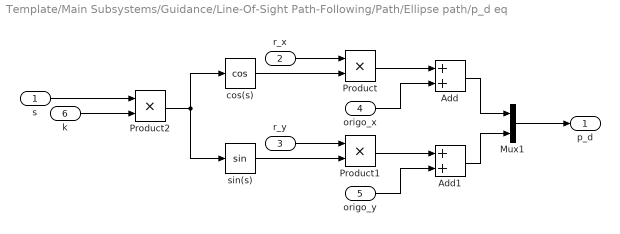
== system Template/Main Subsystems/Guidance/Line-Of-Sight Path-Following/Path/Ellipse path/p_d eq ==
  s : Inport
  r_x : Inport  Port=2
  r_y : Inport  Port=3
  origo_x : Inport  Port=4
  origo_y : Inport  Port=5
  k : Inport  Port=6
  Add : Sum  OutDataType=fixdt(1, 16)  OutScaling=2^-10
  Add1 : Sum  OutDataType=fixdt(1, 16)  OutScaling=2^-10
  Mux1 : Mux  Inputs=2
  Product : Product  OutDataType=fixdt(1, 16)  OutScaling=2^0  RndMeth=Zero
  Product1 : Product  OutDataType=fixdt(1, 16)  OutScaling=2^0  RndMeth=Zero
  Product2 : Product  OutDataType=fixdt(1, 16)  OutScaling=2^0  RndMeth=Zero
  cos(s) : Trigonometry  Operator=cos
  sin(s) : Trigonometry
  p_d : Outport
  wires:
  Product2/1 -> sin(s)/1, cos(s)/1
  k/1 -> Product2/2
  s/1 -> Product2/1
  Add1/1 -> Mux1/2
  Product1/1 -> Add1/1
  Product/1 -> Add/1
  origo_y/1 -> Add1/2
  origo_x/1 -> Add/2
  Mux1/1 -> p_d/1
  r_y/1 -> Product1/1
  r_x/1 -> Product/1
  Add/1 -> Mux1/1
  sin(s)/1 -> Product1/2
  cos(s)/1 -> Product/2

== system Template/Main Subsystems/Guidance/Line-Of-Sight Path-Following/Path/Ellipse path/p_d^s eq ==
  s : Inport
  a : Inport  Port=2
  b : Inport  Port=3
  k : Inport  Port=4
  Gain : Gain  Gain=-1  ParameterDataType=fixdt(1, 16)  ParameterScaling=2^0  OutDataType=fixdt(1, 16)  OutScaling=2^0
  Mux1 : Mux  Inputs=2
  Product : Product  Inputs=3  OutDataType=fixdt(1, 16)  OutScaling=2^0  RndMeth=Zero
  Product1 : Product  Inputs=3  OutDataType=fixdt(1, 16)  OutScaling=2^0  RndMeth=Zero
  Product2 : Product  OutDataType=fixdt(1, 16)  OutScaling=2^0  RndMeth=Zero
  cos(s) : Trigonometry  Operator=cos
  sin(s) : Trigonometry
  p_d^s : Outport
  wires:
  Product2/1 -> sin(s)/1, cos(s)/1
  k/1 -> Product/3, Product1/3, Product2/2
  Mux1/1 -> p_d^s/1
  b/1 -> Product1/1
  a/1 -> Product/1
  Product1/1 -> Mux1/2
  Gain/1 -> Mux1/1
  Product/1 -> Gain/1
  cos(s)/1 -> Product1/2
  sin(s)/1 -> Product/2
  s/1 -> Product2/1

== system Template/Main Subsystems/Guidance/Line-Of-Sight Path-Following/Path/Ellipse path/p_d^s^2 eq ==
  s : Inport
  a : Inport  Port=2
  b : Inport  Port=3
  k : Inport  Port=4
  Gain : Gain  Gain=-1  ParameterDataType=fixdt(1, 16)  ParameterScaling=2^0  OutDataType=fixdt(1, 16)  OutScaling=2^0
  Gain1 : Gain  Gain=-1  ParameterDataType=fixdt(1, 16)  ParameterScaling=2^0  OutDataType=fixdt(1, 16)  OutScaling=2^0
  Math Function : Math  Operator=square  OutDataType=fixdt(1, 16)  OutScaling=2^0  SaturateOnIntegerOverflow=on
  Mux2 : Mux  Inputs=2
  Product : Product  Inputs=3  OutDataType=fixdt(1, 16)  OutScaling=2^0  RndMeth=Zero
  Product1 : Product  Inputs=3  OutDataType=fixdt(1, 16)  OutScaling=2^0  RndMeth=Zero
  Product2 : Product  OutDataType=fixdt(1, 16)  OutScaling=2^0  RndMeth=Zero
  cos(s) : Trigonometry  Operator=cos
  sin(s) : Trigonometry
  p_d^s^2 : Outport
  wires:
  Math Function/1 -> Product/3, Product1/3
  Product2/1 -> sin(s)/1, cos(s)/1
  s/1 -> Product2/1
  k/1 -> Math Function/1, Product2/2
  a/1 -> Product/1
  b/1 -> Product1/1
  Mux2/1 -> p_d^s^2/1
  sin(s)/1 -> Product1/2
  cos(s)/1 -> Product/2
  Gain1/1 -> Mux2/2
  Product1/1 -> Gain1/1
  Gain/1 -> Mux2/1
  Product/1 -> Gain/1

== system Template/Main Subsystems/Guidance/Line-Of-Sight Path-Following/Path/Ellipse path/p_d^s^3 eq ==
  s : Inport
  a : Inport  Port=2
  b : Inport  Port=3
  k : Inport  Port=4
  Constant : Constant  Value=3  OutDataType=fixdt(1, 16)  OutScaling=2^0
  Gain : Gain  Gain=-1  ParameterDataType=fixdt(1, 16)  ParameterScaling=2^0  OutDataType=fixdt(1, 16)  OutScaling=2^0
  Math Function : Math  Operator=pow  OutDataType=fixdt(1, 16)  OutScaling=2^0  SaturateOnIntegerOverflow=on
  Mux3 : Mux  Inputs=2
  Product : Product  Inputs=3  OutDataType=fixdt(1, 16)  OutScaling=2^0  RndMeth=Zero
  Product1 : Product  Inputs=3  OutDataType=fixdt(1, 16)  OutScaling=2^0  RndMeth=Zero
  Product2 : Product  OutDataType=fixdt(1, 16)  OutScaling=2^0  RndMeth=Zero
  cos(s)3 : Trigonometry  Operator=cos
  sin(s)3 : Trigonometry
  p_d^s^3 : Outport
  wires:
  Math Function/1 -> Product/3, Product1/3
  Constant/1 -> Math Function/2
  Product2/1 -> cos(s)3/1, sin(s)3/1
  s/1 -> Product2/1
  k/1 -> Math Function/1, Product2/2
  b/1 -> Product1/1
  a/1 -> Product/1
  sin(s)3/1 -> Product/2
  cos(s)3/1 -> Product1/2
  Product/1 -> Mux3/1
  Mux3/1 -> p_d^s^3/1
  Gain/1 -> Mux3/2
  Product1/1 -> Gain/1

== system Template/Main Subsystems/Guidance/Line-Of-Sight Path-Following/Path/Ellipse path/|p_d^s| eq ==
  p_d^s : Inport
  Product : Product  Multiplication=Matrix(*)  OutDataType=fixdt(1, 16)  OutScaling=2^0  RndMeth=Zero
  Transpose : dspmtrx3/Transpose  SystemSampleTime=-1  Hermitian=off  overflowFlag=off
  sqrt : Math  Operator=sqrt  OutDataType=fixdt(1, 16)  OutScaling=2^0  SaturateOnIntegerOverflow=on
  |p_d^s| : Outport
  wires:
  p_d^s/1 -> Product/2, Transpose/1
  sqrt/1 -> |p_d^s|/1
  Product/1 -> sqrt/1
  Transpose/1 -> Product/1

== system Template/Main Subsystems/Guidance/Line-Of-Sight Path-Following/Path/Path Switch workaround/p_d selcetor ==
  note: Path Selector == 1: Straight path
      | Path Selector == 0: Ellipse path
  Path Selector : Inport  OutDataType=fixdt(1, 16)  OutScaling=2^0
  p_d Straight path : Inport  Port=2  OutDataType=fixdt(1, 16)  OutScaling=2^0
  p_d Ellipse path : Inport  Port=3  OutDataType=fixdt(1, 16)  OutScaling=2^0
  1 - a : Sum  Inputs=+-  OutDataType=fixdt(1, 16)  OutScaling=2^-10
  Add : Sum  OutDataType=fixdt(1, 16)  OutScaling=2^-10
  Constant : Constant  OutDataType=fixdt(1, 16)  OutScaling=2^0
  p_d1 *a : Product  OutDataType=fixdt(1, 16)  OutScaling=2^0  RndMeth=Zero
  p_d2 * (1- a ) : Product  OutDataType=fixdt(1, 16)  OutScaling=2^0  RndMeth=Zero
  p_d : Outport
  wires:
  p_d Ellipse path/1 -> p_d2 * (1- a )/1
  p_d Straight path/1 -> p_d1 *a/1
  Add/1 -> p_d/1
  Path Selector/1 -> p_d1 *a/2, 1 - a/2  "chosen path"
  Constant/1 -> 1 - a/1
  p_d1 *a/1 -> Add/1
  1 - a/1 -> p_d2 * (1- a )/2
  p_d2 * (1- a )/1 -> Add/2

== system Template/Main Subsystems/Guidance/Line-Of-Sight Path-Following/Path/Path Switch workaround/p_d^s selcetor ==
  note: Path Selector == 1: Straight path
      | Path Selector == 0: Ellipse path
  Path Selector : Inport  OutDataType=fixdt(1, 16)  OutScaling=2^0
  p_d^s Straight path : Inport  Port=2  OutDataType=fixdt(1, 16)  OutScaling=2^0
  p_d^s Ellipse path : Inport  Port=3  OutDataType=fixdt(1, 16)  OutScaling=2^0
  Add : Sum  OutDataType=fixdt(1, 16)  OutScaling=2^-10
  Constant : Constant  OutDataType=fixdt(1, 16)  OutScaling=2^0
  Product : Product  OutDataType=fixdt(1, 16)  OutScaling=2^0  RndMeth=Zero
  Product1 : Product  OutDataType=fixdt(1, 16)  OutScaling=2^0  RndMeth=Zero
  Subtract : Sum  Inputs=+-  OutDataType=fixdt(1, 16)  OutScaling=2^-10
  p_d^s : Outport
  wires:
  Product1/1 -> Add/2
  Subtract/1 -> Product1/2
  Product/1 -> Add/1
  Constant/1 -> Subtract/1
  Path Selector/1 -> Subtract/2, Product/2  "chosen path"
  Add/1 -> p_d^s/1
  p_d^s Straight path/1 -> Product/1
  p_d^s Ellipse path/1 -> Product1/1

== system Template/Main Subsystems/Guidance/Line-Of-Sight Path-Following/Path/Path Switch workaround/p_d^s^3 selcetor ==
  note: Path Selector == 1: Straight path
      | Path Selector == 0: Ellipse path
  Path Selector : Inport  OutDataType=fixdt(1, 16)  OutScaling=2^0
  p_d^s^3 Straight path : Inport  Port=2  OutDataType=fixdt(1, 16)  OutScaling=2^0
  p_d^s^3 Ellipse path : Inport  Port=3  OutDataType=fixdt(1, 16)  OutScaling=2^0
  Add : Sum  OutDataType=fixdt(1, 16)  OutScaling=2^-10
  Constant : Constant  OutDataType=fixdt(1, 16)  OutScaling=2^0
  Product : Product  OutDataType=fixdt(1, 16)  OutScaling=2^0  RndMeth=Zero
  Product1 : Product  OutDataType=fixdt(1, 16)  OutScaling=2^0  RndMeth=Zero
  Subtract : Sum  Inputs=+-  OutDataType=fixdt(1, 16)  OutScaling=2^-10
  "p_d^s^3 " : Outport
  wires:
  Product1/1 -> Add/2
  Subtract/1 -> Product1/2
  Product/1 -> Add/1
  Constant/1 -> Subtract/1
  Path Selector/1 -> Subtract/2, Product/2  "chosen path"
  Add/1 -> "p_d^s^3 "/1
  p_d^s^3 Straight path/1 -> Product/1
  p_d^s^3 Ellipse path/1 -> Product1/1

== system Template/Main Subsystems/Guidance/Line-Of-Sight Path-Following/Path/Path Switch workaround/p_ds^2 selcetor ==
  note: Path Selector == 1: Straight path
      | Path Selector == 0: Ellipse path
  Path Selector : Inport  OutDataType=fixdt(1, 16)  OutScaling=2^0
  p_ds^2  Straight path : Inport  Port=2  OutDataType=fixdt(1, 16)  OutScaling=2^0
  p_ds^2  Ellipse path : Inport  Port=3  OutDataType=fixdt(1, 16)  OutScaling=2^0
  Add : Sum  OutDataType=fixdt(1, 16)  OutScaling=2^-10
  Constant : Constant  OutDataType=fixdt(1, 16)  OutScaling=2^0
  Product : Product  OutDataType=fixdt(1, 16)  OutScaling=2^0  RndMeth=Zero
  Product1 : Product  OutDataType=fixdt(1, 16)  OutScaling=2^0  RndMeth=Zero
  Subtract : Sum  Inputs=+-  OutDataType=fixdt(1, 16)  OutScaling=2^-10
  "p_ds^2 " : Outport
  wires:
  Product1/1 -> Add/2
  Subtract/1 -> Product1/2
  Product/1 -> Add/1
  Constant/1 -> Subtract/1
  Path Selector/1 -> Subtract/2, Product/2  "chosen path"
  Add/1 -> "p_ds^2 "/1
  p_ds^2  Straight path/1 -> Product/1
  p_ds^2  Ellipse path/1 -> Product1/1

== system Template/Main Subsystems/Guidance/Line-Of-Sight Path-Following/Path/Path Switch workaround/|p_d^s| selcetor ==
  note: Path Selector == 1: Straight path
      | Path Selector == 0: Ellipse path
  Path Selector : Inport  OutDataType=fixdt(1, 16)  OutScaling=2^0
  |p_d^s| Straight path : Inport  Port=2  OutDataType=fixdt(1, 16)  OutScaling=2^0
  |p_d^s| Ellipse path : Inport  Port=3  OutDataType=fixdt(1, 16)  OutScaling=2^0
  Add : Sum  OutDataType=fixdt(1, 16)  OutScaling=2^-10
  Constant : Constant  OutDataType=fixdt(1, 16)  OutScaling=2^0
  Product : Product  OutDataType=fixdt(1, 16)  OutScaling=2^0  RndMeth=Zero
  Product1 : Product  OutDataType=fixdt(1, 16)  OutScaling=2^0  RndMeth=Zero
  Subtract : Sum  Inputs=+-  OutDataType=fixdt(1, 16)  OutScaling=2^-10
  |p_d^s| : Outport
  wires:
  Product1/1 -> Add/2
  Subtract/1 -> Product1/2
  Product/1 -> Add/1
  Constant/1 -> Subtract/1
  Path Selector/1 -> Subtract/2, Product/2  "chosen path"
  Add/1 -> |p_d^s|/1
  |p_d^s| Straight path/1 -> Product/1
  |p_d^s| Ellipse path/1 -> Product1/1

== system Template/Main Subsystems/Guidance/Line-Of-Sight Path-Following/Path/Straight path/p_d eq ==
  s : Inport
  x_1 : Inport  Port=2
  y_1 : Inport  Port=3
  x_2 : Inport  Port=4
  y_2 : Inport  Port=5
  (x_2 - x_1) * s : Product  OutDataType=fixdt(1, 16)  OutScaling=2^0  RndMeth=Zero
  (x_2 - x_1) * s + x_1 : Sum  OutDataType=fixdt(1, 16)  OutScaling=2^-10
  (y_2 - y_1) * s : Product  OutDataType=fixdt(1, 16)  OutScaling=2^0  RndMeth=Zero
  (y_2 - y_1) * s + y_1 : Sum  OutDataType=fixdt(1, 16)  OutScaling=2^-10
  Mux1 : Mux  Inputs=2
  x_2 - x_1 : Sum  Inputs=+-  OutDataType=fixdt(1, 16)  OutScaling=2^-10
  y_2 - y_1 : Sum  Inputs=+-  OutDataType=fixdt(1, 16)  OutScaling=2^-10
  p_d : Outport
  wires:
  Mux1/1 -> p_d/1
  y_1/1 -> (y_2 - y_1) * s + y_1/2, y_2 - y_1/2
  y_2/1 -> y_2 - y_1/1
  x_1/1 -> (x_2 - x_1) * s + x_1/2, x_2 - x_1/2
  x_2/1 -> x_2 - x_1/1
  s/1 -> (y_2 - y_1) * s/2, (x_2 - x_1) * s/2
  y_2 - y_1/1 -> (y_2 - y_1) * s/1
  x_2 - x_1/1 -> (x_2 - x_1) * s/1
  (y_2 - y_1) * s/1 -> (y_2 - y_1) * s + y_1/1
  (x_2 - x_1) * s/1 -> (x_2 - x_1) * s + x_1/1
  (y_2 - y_1) * s + y_1/1 -> Mux1/2
  (x_2 - x_1) * s + x_1/1 -> Mux1/1

== system Template/Main Subsystems/Guidance/Line-Of-Sight Path-Following/Path/Straight path/p_d^s eq ==
  x_1 : Inport
  y_1 : Inport  Port=2
  x_2 : Inport  Port=3
  y_2 : Inport  Port=4
  Mux1 : Mux  Inputs=2
  x_2 - x_1 : Sum  Inputs=+-  OutDataType=fixdt(1, 16)  OutScaling=2^-10
  y_2 - y_1 : Sum  Inputs=+-  OutDataType=fixdt(1, 16)  OutScaling=2^-10
  p_d^s : Outport
  wires:
  y_1/1 -> y_2 - y_1/2
  y_2/1 -> y_2 - y_1/1
  x_1/1 -> x_2 - x_1/2
  x_2/1 -> x_2 - x_1/1
  y_2 - y_1/1 -> Mux1/2
  x_2 - x_1/1 -> Mux1/1
  Mux1/1 -> p_d^s/1

== system Template/Main Subsystems/Guidance/Line-Of-Sight Path-Following/Path/Straight path/|p_d^s| eq ==
  p_d^s : Inport
  Product : Product  Multiplication=Matrix(*)  OutDataType=fixdt(1, 16)  OutScaling=2^0  RndMeth=Zero
  p_d^s^T : dspmtrx3/Transpose  SystemSampleTime=-1  Hermitian=off  overflowFlag=off
  sqrt : Math  Operator=sqrt  OutDataType=fixdt(1, 16)  OutScaling=2^0  SaturateOnIntegerOverflow=on
  |p_d^s| : Outport
  wires:
  p_d^s/1 -> Product/2, p_d^s^T/1
  sqrt/1 -> |p_d^s|/1
  Product/1 -> sqrt/1
  p_d^s^T/1 -> Product/1
